simulink model "model3"  (R2022a)
settings: Solver=VariableStepAuto  StartTime=0.0  StopTime=200  RelTol=1e-3
settings Model: Creator=tano-  LastModifiedBy=tano-

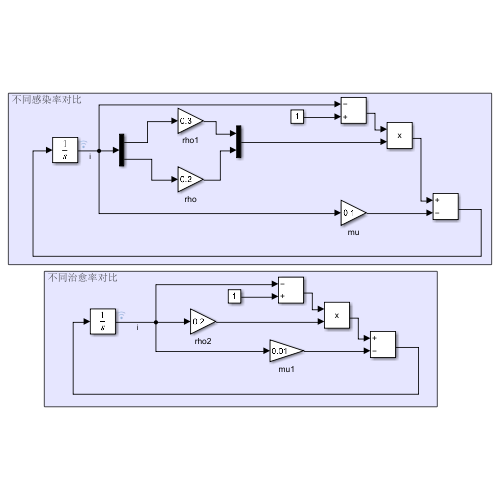
[thumbnail: Simulink's stored preview of the top-level diagram]
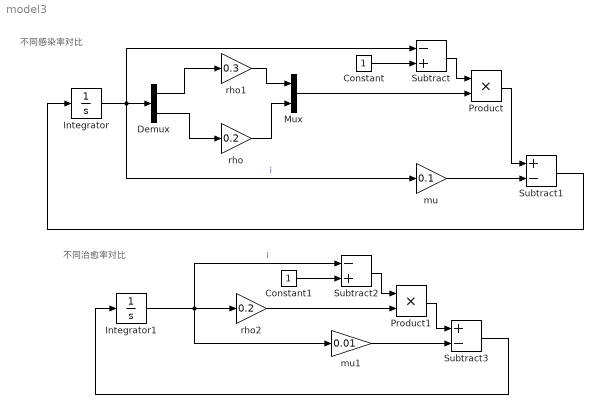
== system model3 ==
  note: 不同治愈率对比
  note: 不同感染率对比
  Constant : Constant
  Constant1 : Constant
  Demux : Demux  Outputs=2
  Integrator : Integrator  InitialCondition=[0.0001 0.0001]
  Integrator1 : Integrator  InitialCondition=0.0001
  Mux : Mux  Inputs=2
  Product : Product
  Product1 : Product
  Subtract : Sum  Inputs=-+
  Subtract1 : Sum  Inputs=+-
  Subtract2 : Sum  Inputs=-+
  Subtract3 : Sum  Inputs=+-
  mu : Gain  Gain=0.1
  mu1 : Gain  Gain=0.01
  rho : Gain  Gain=0.2
  rho1 : Gain  Gain=0.3
  rho2 : Gain  Gain=0.2
  wires:
  Subtract/1 -> Product/1
  Mux/1 -> Product/2
  rho/1 -> Mux/2
  Integrator/1 -> Subtract/1, Demux/1, mu/1  "i"
  Demux/2 -> rho/1
  rho1/1 -> Mux/1
  Demux/1 -> rho1/1
  Constant/1 -> Subtract/2
  mu/1 -> Subtract1/2
  Product/1 -> Subtract1/1
  Subtract1/1 -> Integrator/1
  Subtract3/1 -> Integrator1/1
  Product1/1 -> Subtract3/1
  mu1/1 -> Subtract3/2
  Constant1/1 -> Subtract2/2
  Integrator1/1 -> mu1/1, Subtract2/1, rho2/1  "i"
  Subtract2/1 -> Product1/1
  rho2/1 -> Product1/2
